simulink model "g_s_cl4"  (Simulink 5.0)
settings: Solver=ode45  StartTime=t_init  StopTime=t_final  RelTol=1e-3
values from neighbouring files (symbols this model uses):
  C = A+B    [poladd.m]
undefined symbols (not defined in the file or in its folder): D, den, num, Rb, Rf, Sb, Sf, st, st1, Ts
settings Model: Creator=kannan  LastModifiedBy=kannan  ExtModeAutoUpdateStatusClock=off

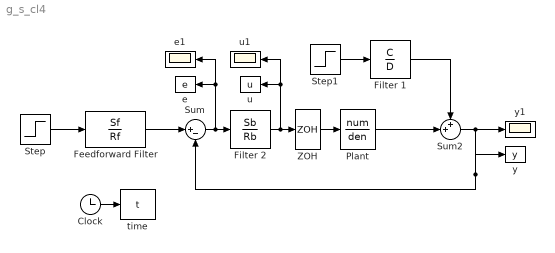
== system g_s_cl4 ==
  " Filter 2" : DiscreteFilter  Numerator=Sb  Denominator=Rb  SampleTime=Ts
  Clock : Clock
      settings: Decimation=10
  Feedforward Filter : DiscreteFilter  Numerator=Sf  Denominator=Rf  SampleTime=Ts
  Filter 1 : DiscreteFilter  Numerator=C  Denominator=D  SampleTime=Ts
  Plant : TransferFcn  Numerator=num  Denominator=den
  Step : Step  Time=0  After=st  SampleTime=Ts
  Step1 : Step  Time=0  After=st1  SampleTime=Ts
  Sum : Sum  Inputs=|+-  SaturateOnIntegerOverflow=on
  Sum2 : Sum  Inputs=++|  SaturateOnIntegerOverflow=on
  ZOH : ZeroOrderHold  SampleTime=Ts
  e : ToWorkspace  VariableName=e  SampleTime=Ts  SaveFormat=Array
  e1 : Scope
      settings: YMin=-6e+164  YMax=1.02293e+149  SaveName=ScopeData2
  time : ToWorkspace  VariableName=t  SampleTime=Ts  SaveFormat=Array
  u : ToWorkspace  VariableName=u  SampleTime=Ts  SaveFormat=Array
  u1 : Scope
      settings: YMin=-6e+164  YMax=1.02293e+149
  y : ToWorkspace  VariableName=y  SampleTime=Ts  SaveFormat=Array
  y1 : Scope
      settings: YMin=-6e+164  YMax=1.02293e+149
  wires:
  Feedforward Filter/1 -> Sum/1
  Clock/1 -> time/1
  Plant/1 -> Sum2/2
  Filter 1/1 -> Sum2/1
  Step1/1 -> Filter 1/1
  Sum2/1 -> y1/1, y/1, Sum/2
  Sum/1 -> " Filter 2"/1, e/1, e1/1
  " Filter 2"/1 -> u1/1, u/1, ZOH/1
  ZOH/1 -> Plant/1
  Step/1 -> Feedforward Filter/1
